simulink model "TST_PthLead_TrqCalc"  (R2016b)
settings: Solver=FixedStepDiscrete  StartTime=0.0  StopTime=simTime  FixedStep=sampleTime  RelTol=1e-3
values from neighbouring files (symbols this model uses):
  testCase = 1    [initTST_PthLead_TrqCalc_001.m]    (also in initTST_PthLead_TrqCalc_002.m = 2; initTST_PthLead_TrqCalc_003.m = 3)
libraries: simulink x13, UnitTest_Lib x9
settings Model: Creator=zhengjinyan  LastModifiedBy=zhengjinyan
settings DebuggingCC: SignalRangeChecking=error

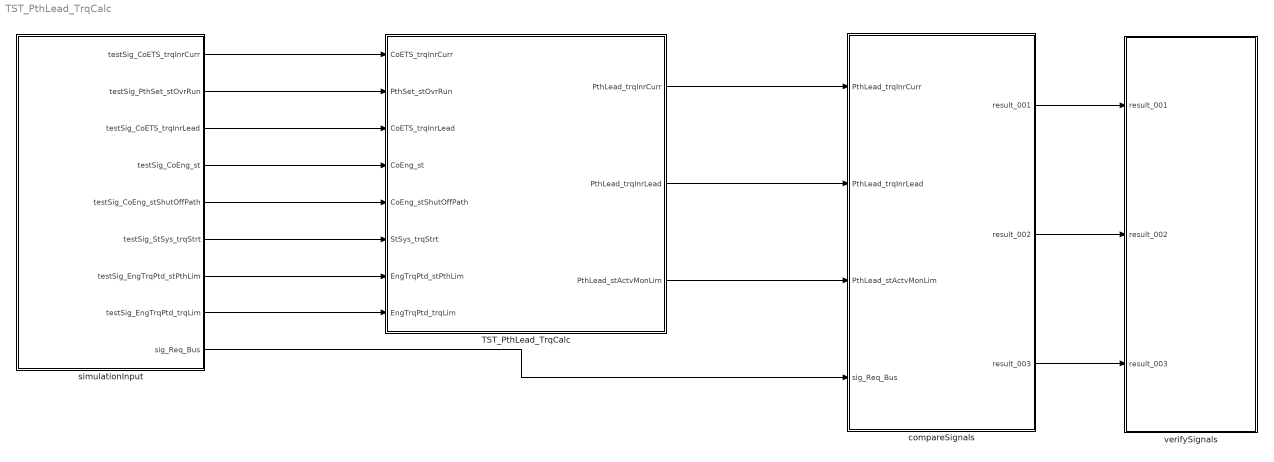
== system TST_PthLead_TrqCalc ==
  TST_PthLead_TrqCalc : Subsystem
  compareSignals : Subsystem
  simulationInput : Subsystem
  verifySignals : Subsystem
  wires:
  simulationInput/1(testSig_CoETS_trqInrCurr) -> TST_PthLead_TrqCalc/1(CoETS_trqInrCurr)
  simulationInput/2(testSig_PthSet_stOvrRun) -> TST_PthLead_TrqCalc/2(PthSet_stOvrRun)
  simulationInput/3(testSig_CoETS_trqInrLead) -> TST_PthLead_TrqCalc/3(CoETS_trqInrLead)
  simulationInput/4(testSig_CoEng_st) -> TST_PthLead_TrqCalc/4(CoEng_st)
  simulationInput/5(testSig_CoEng_stShutOffPath) -> TST_PthLead_TrqCalc/5(CoEng_stShutOffPath)
  simulationInput/6(testSig_StSys_trqStrt) -> TST_PthLead_TrqCalc/6(StSys_trqStrt)
  simulationInput/7(testSig_EngTrqPtd_stPthLim) -> TST_PthLead_TrqCalc/7(EngTrqPtd_stPthLim)
  simulationInput/8(testSig_EngTrqPtd_trqLim) -> TST_PthLead_TrqCalc/8(EngTrqPtd_trqLim)
  TST_PthLead_TrqCalc/1(PthLead_trqInrCurr) -> compareSignals/1(PthLead_trqInrCurr)
  TST_PthLead_TrqCalc/2(PthLead_trqInrLead) -> compareSignals/2(PthLead_trqInrLead)
  TST_PthLead_TrqCalc/3(PthLead_stActvMonLim) -> compareSignals/3(PthLead_stActvMonLim)
  simulationInput/9(sig_Req_Bus) -> compareSignals/4(sig_Req_Bus)
  compareSignals/1(result_001) -> verifySignals/1(result_001)
  compareSignals/2(result_002) -> verifySignals/2(result_002)
  compareSignals/3(result_003) -> verifySignals/3(result_003)

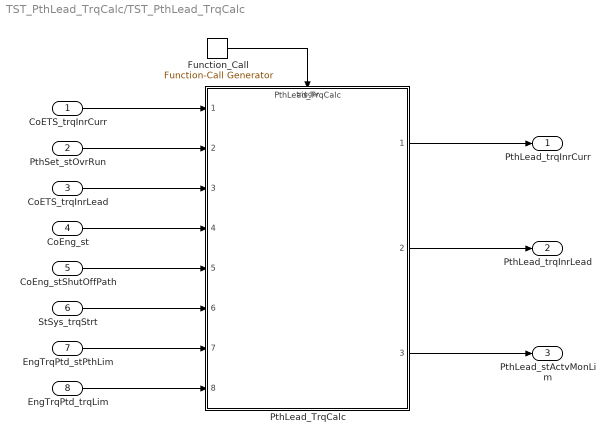
== system TST_PthLead_TrqCalc/TST_PthLead_TrqCalc ==
  CoETS_trqInrCurr : Inport
  PthSet_stOvrRun : Inport  Port=2
  CoETS_trqInrLead : Inport  Port=3
  CoEng_st : Inport  Port=4
  CoEng_stShutOffPath : Inport  Port=5
  StSys_trqStrt : Inport  Port=6
  EngTrqPtd_stPthLim : Inport  Port=7
  EngTrqPtd_trqLim : Inport  Port=8
  Function_Call : simulink/Ports & Subsystems/Function-Call Generator  sample_time=sampleTime  numberOfIterations=1
  PthLead_TrqCalc : ModelReference  ModelNameDialog=PthLead_TrqCalc  SimulationMode=Normal  ModelReferenceVersion=1.4  TriggerPortName=function  TriggerPortTriggerType=function-call  TriggerPortStatesWhenEnabling=held
  PthLead_trqInrCurr : Outport
  PthLead_trqInrLead : Outport  Port=2
  PthLead_stActvMonLim : Outport  Port=3
  wires:
  Function_Call/1 -> PthLead_TrqCalc/Trigger
  CoETS_trqInrCurr/1 -> PthLead_TrqCalc/1
  PthSet_stOvrRun/1 -> PthLead_TrqCalc/2
  CoETS_trqInrLead/1 -> PthLead_TrqCalc/3
  CoEng_st/1 -> PthLead_TrqCalc/4
  CoEng_stShutOffPath/1 -> PthLead_TrqCalc/5
  StSys_trqStrt/1 -> PthLead_TrqCalc/6
  EngTrqPtd_stPthLim/1 -> PthLead_TrqCalc/7
  EngTrqPtd_trqLim/1 -> PthLead_TrqCalc/8
  PthLead_TrqCalc/1 -> PthLead_trqInrCurr/1
  PthLead_TrqCalc/2 -> PthLead_trqInrLead/1
  PthLead_TrqCalc/3 -> PthLead_stActvMonLim/1

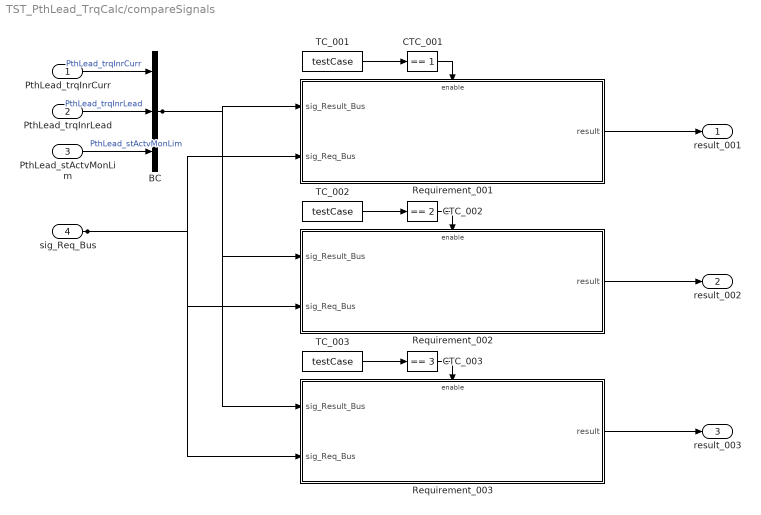
== system TST_PthLead_TrqCalc/compareSignals ==
  PthLead_trqInrCurr : Inport
  PthLead_trqInrLead : Inport  Port=2
  PthLead_stActvMonLim : Inport  Port=3
  sig_Req_Bus : Inport  Port=4
  BC : BusCreator  Inputs=3
  CTC_001 : simulink/Logic and Bit Operations/Compare To Constant  relop===  const=1  OutDataTypeStr=boolean
  CTC_002 : simulink/Logic and Bit Operations/Compare To Constant  relop===  const=2  OutDataTypeStr=boolean
  CTC_003 : simulink/Logic and Bit Operations/Compare To Constant  relop===  const=3  OutDataTypeStr=boolean
  Requirement_001 : Subsystem
  Requirement_002 : Subsystem
  Requirement_003 : Subsystem
  TC_001 : Constant  Value=testCase
  TC_002 : Constant  Value=testCase
  TC_003 : Constant  Value=testCase
  result_001 : Outport
  result_002 : Outport  Port=2
  result_003 : Outport  Port=3
  wires:
  PthLead_trqInrCurr/1 -> BC/1  "PthLead_trqInrCurr"
  PthLead_trqInrLead/1 -> BC/2  "PthLead_trqInrLead"
  PthLead_stActvMonLim/1 -> BC/3  "PthLead_stActvMonLim"
  TC_001/1 -> CTC_001/1
  CTC_001/1 -> Requirement_001/Enable
  sig_Req_Bus/1 -> Requirement_001/2(sig_Req_Bus), Requirement_002/2(sig_Req_Bus), Requirement_003/2(sig_Req_Bus)
  BC/1 -> Requirement_001/1(sig_Result_Bus), Requirement_002/1(sig_Result_Bus), Requirement_003/1(sig_Result_Bus)
  Requirement_001/1(result) -> result_001/1
  TC_002/1 -> CTC_002/1
  CTC_002/1 -> Requirement_002/Enable
  Requirement_002/1(result) -> result_002/1
  TC_003/1 -> CTC_003/1
  CTC_003/1 -> Requirement_003/Enable
  Requirement_003/1(result) -> result_003/1

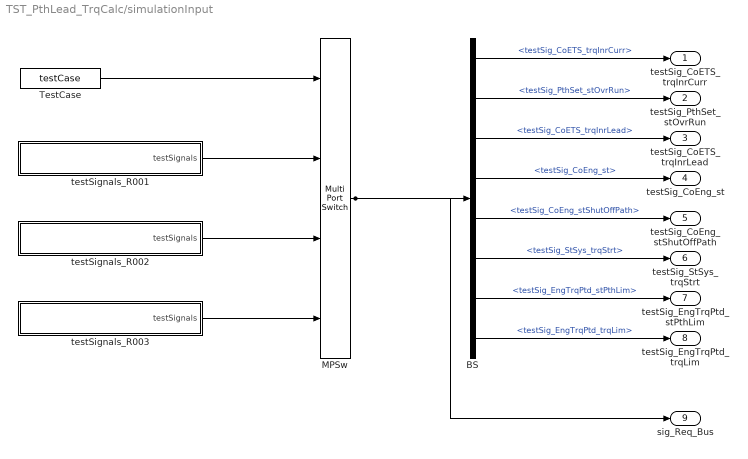
== system TST_PthLead_TrqCalc/simulationInput ==
  BS : BusSelector  OutputSignals=testSig_CoETS_trqInrCurr,testSig_PthSet_stOvrRun,testSig_CoETS_trqInrLead,testSig_CoEng_st,testSig_CoEng_stShutOffPath,testSig_StSys_trqStrt,testSig_EngTrqPtd_stPthLim,testSig_EngTrqPtd_trqLim
  MPSw : MultiPortSwitch  SaturateOnIntegerOverflow=on  InputSameDT=on
  TestCase : Constant  Value=testCase
  testSignals_R001 : Subsystem
  testSignals_R002 : Subsystem
  testSignals_R003 : Subsystem
  testSig_CoETS_trqInrCurr : Outport
  testSig_PthSet_stOvrRun : Outport  Port=2
  testSig_CoETS_trqInrLead : Outport  Port=3
  testSig_CoEng_st : Outport  Port=4
  testSig_CoEng_stShutOffPath : Outport  Port=5
  testSig_StSys_trqStrt : Outport  Port=6
  testSig_EngTrqPtd_stPthLim : Outport  Port=7
  testSig_EngTrqPtd_trqLim : Outport  Port=8
  sig_Req_Bus : Outport  Port=9
  wires:
  BS/1 -> testSig_CoETS_trqInrCurr/1  "<testSig_CoETS_trqInrCurr>"
  BS/2 -> testSig_PthSet_stOvrRun/1  "<testSig_PthSet_stOvrRun>"
  BS/3 -> testSig_CoETS_trqInrLead/1  "<testSig_CoETS_trqInrLead>"
  BS/4 -> testSig_CoEng_st/1  "<testSig_CoEng_st>"
  BS/5 -> testSig_CoEng_stShutOffPath/1  "<testSig_CoEng_stShutOffPath>"
  BS/6 -> testSig_StSys_trqStrt/1  "<testSig_StSys_trqStrt>"
  BS/7 -> testSig_EngTrqPtd_stPthLim/1  "<testSig_EngTrqPtd_stPthLim>"
  BS/8 -> testSig_EngTrqPtd_trqLim/1  "<testSig_EngTrqPtd_trqLim>"
  MPSw/1 -> BS/1, sig_Req_Bus/1
  TestCase/1 -> MPSw/1
  testSignals_R001/1(testSignals) -> MPSw/2
  testSignals_R002/1(testSignals) -> MPSw/3
  testSignals_R003/1(testSignals) -> MPSw/4

== system TST_PthLead_TrqCalc/verifySignals ==
  result_001 : Inport
  result_002 : Inport  Port=2
  result_003 : Inport  Port=3
  Assertion_001 : Assertion  Enabled=off
  Assertion_002 : Assertion  Enabled=off
  Assertion_003 : Assertion  Enabled=off
  wires:
  result_001/1 -> Assertion_001/1
  result_002/1 -> Assertion_002/1
  result_003/1 -> Assertion_003/1

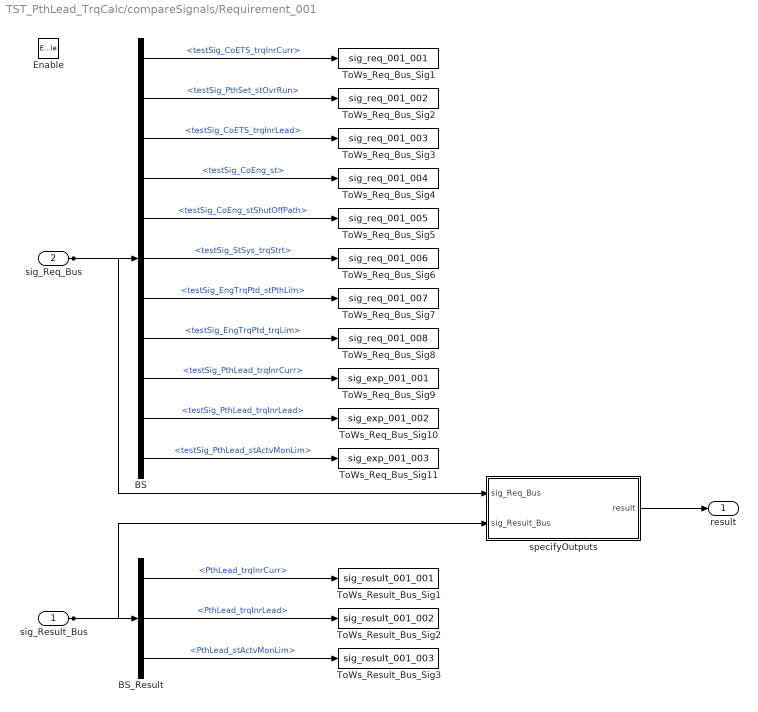
== system TST_PthLead_TrqCalc/compareSignals/Requirement_001 ==
  sig_Result_Bus : Inport
  sig_Req_Bus : Inport  Port=2
  Enable : EnablePort
  BS : BusSelector  OutputSignals=testSig_CoETS_trqInrCurr,testSig_PthSet_stOvrRun,testSig_CoETS_trqInrLead,testSig_CoEng_st,testSig_CoEng_stShutOffPath,testSig_StSys_trqStrt,testSig_EngTrqPtd_stPthLim,testSig_EngTrqPtd_trqLim,testSig_PthLead_trqInrCurr,testSig_PthLead_trqInrLead,testSig_PthLead_stActvMonLim
  BS_Result : BusSelector  OutputSignals=PthLead_trqInrCurr,PthLead_trqInrLead,PthLead_stActvMonLim
  ToWs_Req_Bus_Sig1 : ToWorkspace  VariableName=sig_req_001_001  SaveFormat=Structure With Time
  ToWs_Req_Bus_Sig10 : ToWorkspace  VariableName=sig_exp_001_002  SaveFormat=Structure With Time
  ToWs_Req_Bus_Sig11 : ToWorkspace  VariableName=sig_exp_001_003  SaveFormat=Structure With Time
  ToWs_Req_Bus_Sig2 : ToWorkspace  VariableName=sig_req_001_002  SaveFormat=Structure With Time
  ToWs_Req_Bus_Sig3 : ToWorkspace  VariableName=sig_req_001_003  SaveFormat=Structure With Time
  ToWs_Req_Bus_Sig4 : ToWorkspace  VariableName=sig_req_001_004  SaveFormat=Structure With Time
  ToWs_Req_Bus_Sig5 : ToWorkspace  VariableName=sig_req_001_005  SaveFormat=Structure With Time
  ToWs_Req_Bus_Sig6 : ToWorkspace  VariableName=sig_req_001_006  SaveFormat=Structure With Time
  ToWs_Req_Bus_Sig7 : ToWorkspace  VariableName=sig_req_001_007  SaveFormat=Structure With Time
  ToWs_Req_Bus_Sig8 : ToWorkspace  VariableName=sig_req_001_008  SaveFormat=Structure With Time
  ToWs_Req_Bus_Sig9 : ToWorkspace  VariableName=sig_exp_001_001  SaveFormat=Structure With Time
  ToWs_Result_Bus_Sig1 : ToWorkspace  VariableName=sig_result_001_001  SaveFormat=Structure With Time
  ToWs_Result_Bus_Sig2 : ToWorkspace  VariableName=sig_result_001_002  SaveFormat=Structure With Time
  ToWs_Result_Bus_Sig3 : ToWorkspace  VariableName=sig_result_001_003  SaveFormat=Structure With Time
  specifyOutputs : Subsystem
  result : Outport
  wires:
  sig_Req_Bus/1 -> BS/1, specifyOutputs/1(sig_Req_Bus)
  BS/1 -> ToWs_Req_Bus_Sig1/1  "<testSig_CoETS_trqInrCurr>"
  BS/2 -> ToWs_Req_Bus_Sig2/1  "<testSig_PthSet_stOvrRun>"
  BS/3 -> ToWs_Req_Bus_Sig3/1  "<testSig_CoETS_trqInrLead>"
  BS/4 -> ToWs_Req_Bus_Sig4/1  "<testSig_CoEng_st>"
  BS/5 -> ToWs_Req_Bus_Sig5/1  "<testSig_CoEng_stShutOffPath>"
  BS/6 -> ToWs_Req_Bus_Sig6/1  "<testSig_StSys_trqStrt>"
  BS/7 -> ToWs_Req_Bus_Sig7/1  "<testSig_EngTrqPtd_stPthLim>"
  BS/8 -> ToWs_Req_Bus_Sig8/1  "<testSig_EngTrqPtd_trqLim>"
  BS/9 -> ToWs_Req_Bus_Sig9/1  "<testSig_PthLead_trqInrCurr>"
  BS/10 -> ToWs_Req_Bus_Sig10/1  "<testSig_PthLead_trqInrLead>"
  BS/11 -> ToWs_Req_Bus_Sig11/1  "<testSig_PthLead_stActvMonLim>"
  sig_Result_Bus/1 -> BS_Result/1, specifyOutputs/2(sig_Result_Bus)
  BS_Result/1 -> ToWs_Result_Bus_Sig1/1  "<PthLead_trqInrCurr>"
  BS_Result/2 -> ToWs_Result_Bus_Sig2/1  "<PthLead_trqInrLead>"
  BS_Result/3 -> ToWs_Result_Bus_Sig3/1  "<PthLead_stActvMonLim>"
  specifyOutputs/1(result) -> result/1

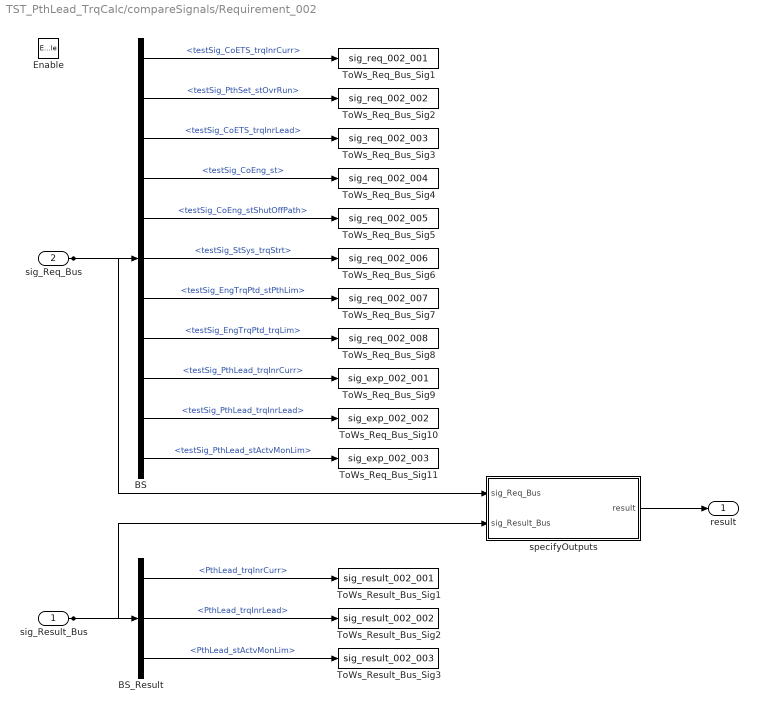
== system TST_PthLead_TrqCalc/compareSignals/Requirement_002 ==
  sig_Result_Bus : Inport
  sig_Req_Bus : Inport  Port=2
  Enable : EnablePort
  BS : BusSelector  OutputSignals=testSig_CoETS_trqInrCurr,testSig_PthSet_stOvrRun,testSig_CoETS_trqInrLead,testSig_CoEng_st,testSig_CoEng_stShutOffPath,testSig_StSys_trqStrt,testSig_EngTrqPtd_stPthLim,testSig_EngTrqPtd_trqLim,testSig_PthLead_trqInrCurr,testSig_PthLead_trqInrLead,testSig_PthLead_stActvMonLim
  BS_Result : BusSelector  OutputSignals=PthLead_trqInrCurr,PthLead_trqInrLead,PthLead_stActvMonLim
  ToWs_Req_Bus_Sig1 : ToWorkspace  VariableName=sig_req_002_001  SaveFormat=Structure With Time
  ToWs_Req_Bus_Sig10 : ToWorkspace  VariableName=sig_exp_002_002  SaveFormat=Structure With Time
  ToWs_Req_Bus_Sig11 : ToWorkspace  VariableName=sig_exp_002_003  SaveFormat=Structure With Time
  ToWs_Req_Bus_Sig2 : ToWorkspace  VariableName=sig_req_002_002  SaveFormat=Structure With Time
  ToWs_Req_Bus_Sig3 : ToWorkspace  VariableName=sig_req_002_003  SaveFormat=Structure With Time
  ToWs_Req_Bus_Sig4 : ToWorkspace  VariableName=sig_req_002_004  SaveFormat=Structure With Time
  ToWs_Req_Bus_Sig5 : ToWorkspace  VariableName=sig_req_002_005  SaveFormat=Structure With Time
  ToWs_Req_Bus_Sig6 : ToWorkspace  VariableName=sig_req_002_006  SaveFormat=Structure With Time
  ToWs_Req_Bus_Sig7 : ToWorkspace  VariableName=sig_req_002_007  SaveFormat=Structure With Time
  ToWs_Req_Bus_Sig8 : ToWorkspace  VariableName=sig_req_002_008  SaveFormat=Structure With Time
  ToWs_Req_Bus_Sig9 : ToWorkspace  VariableName=sig_exp_002_001  SaveFormat=Structure With Time
  ToWs_Result_Bus_Sig1 : ToWorkspace  VariableName=sig_result_002_001  SaveFormat=Structure With Time
  ToWs_Result_Bus_Sig2 : ToWorkspace  VariableName=sig_result_002_002  SaveFormat=Structure With Time
  ToWs_Result_Bus_Sig3 : ToWorkspace  VariableName=sig_result_002_003  SaveFormat=Structure With Time
  specifyOutputs : Subsystem
  result : Outport
  wires:
  sig_Req_Bus/1 -> BS/1, specifyOutputs/1(sig_Req_Bus)
  BS/1 -> ToWs_Req_Bus_Sig1/1  "<testSig_CoETS_trqInrCurr>"
  BS/2 -> ToWs_Req_Bus_Sig2/1  "<testSig_PthSet_stOvrRun>"
  BS/3 -> ToWs_Req_Bus_Sig3/1  "<testSig_CoETS_trqInrLead>"
  BS/4 -> ToWs_Req_Bus_Sig4/1  "<testSig_CoEng_st>"
  BS/5 -> ToWs_Req_Bus_Sig5/1  "<testSig_CoEng_stShutOffPath>"
  BS/6 -> ToWs_Req_Bus_Sig6/1  "<testSig_StSys_trqStrt>"
  BS/7 -> ToWs_Req_Bus_Sig7/1  "<testSig_EngTrqPtd_stPthLim>"
  BS/8 -> ToWs_Req_Bus_Sig8/1  "<testSig_EngTrqPtd_trqLim>"
  BS/9 -> ToWs_Req_Bus_Sig9/1  "<testSig_PthLead_trqInrCurr>"
  BS/10 -> ToWs_Req_Bus_Sig10/1  "<testSig_PthLead_trqInrLead>"
  BS/11 -> ToWs_Req_Bus_Sig11/1  "<testSig_PthLead_stActvMonLim>"
  sig_Result_Bus/1 -> BS_Result/1, specifyOutputs/2(sig_Result_Bus)
  BS_Result/1 -> ToWs_Result_Bus_Sig1/1  "<PthLead_trqInrCurr>"
  BS_Result/2 -> ToWs_Result_Bus_Sig2/1  "<PthLead_trqInrLead>"
  BS_Result/3 -> ToWs_Result_Bus_Sig3/1  "<PthLead_stActvMonLim>"
  specifyOutputs/1(result) -> result/1

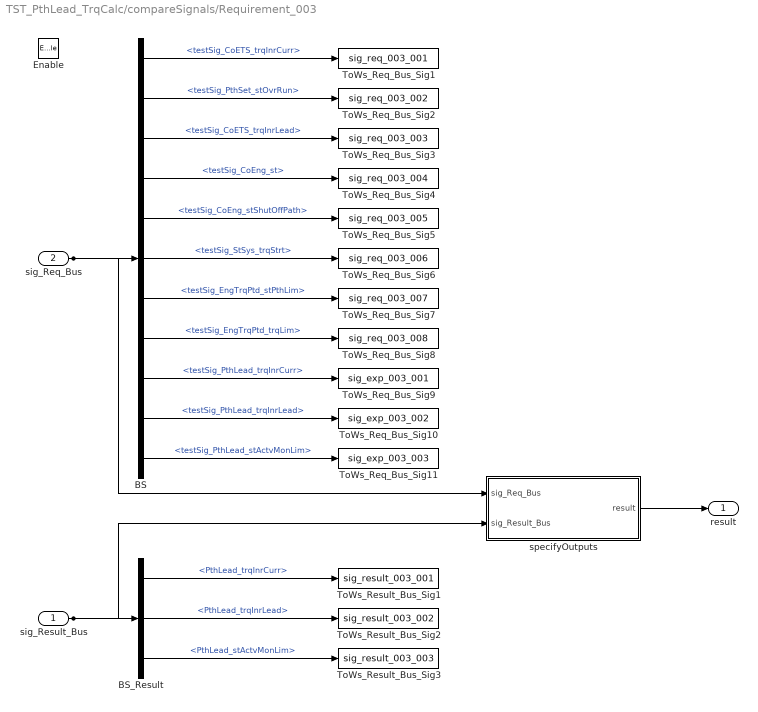
== system TST_PthLead_TrqCalc/compareSignals/Requirement_003 ==
  sig_Result_Bus : Inport
  sig_Req_Bus : Inport  Port=2
  Enable : EnablePort
  BS : BusSelector  OutputSignals=testSig_CoETS_trqInrCurr,testSig_PthSet_stOvrRun,testSig_CoETS_trqInrLead,testSig_CoEng_st,testSig_CoEng_stShutOffPath,testSig_StSys_trqStrt,testSig_EngTrqPtd_stPthLim,testSig_EngTrqPtd_trqLim,testSig_PthLead_trqInrCurr,testSig_PthLead_trqInrLead,testSig_PthLead_stActvMonLim
  BS_Result : BusSelector  OutputSignals=PthLead_trqInrCurr,PthLead_trqInrLead,PthLead_stActvMonLim
  ToWs_Req_Bus_Sig1 : ToWorkspace  VariableName=sig_req_003_001  SaveFormat=Structure With Time
  ToWs_Req_Bus_Sig10 : ToWorkspace  VariableName=sig_exp_003_002  SaveFormat=Structure With Time
  ToWs_Req_Bus_Sig11 : ToWorkspace  VariableName=sig_exp_003_003  SaveFormat=Structure With Time
  ToWs_Req_Bus_Sig2 : ToWorkspace  VariableName=sig_req_003_002  SaveFormat=Structure With Time
  ToWs_Req_Bus_Sig3 : ToWorkspace  VariableName=sig_req_003_003  SaveFormat=Structure With Time
  ToWs_Req_Bus_Sig4 : ToWorkspace  VariableName=sig_req_003_004  SaveFormat=Structure With Time
  ToWs_Req_Bus_Sig5 : ToWorkspace  VariableName=sig_req_003_005  SaveFormat=Structure With Time
  ToWs_Req_Bus_Sig6 : ToWorkspace  VariableName=sig_req_003_006  SaveFormat=Structure With Time
  ToWs_Req_Bus_Sig7 : ToWorkspace  VariableName=sig_req_003_007  SaveFormat=Structure With Time
  ToWs_Req_Bus_Sig8 : ToWorkspace  VariableName=sig_req_003_008  SaveFormat=Structure With Time
  ToWs_Req_Bus_Sig9 : ToWorkspace  VariableName=sig_exp_003_001  SaveFormat=Structure With Time
  ToWs_Result_Bus_Sig1 : ToWorkspace  VariableName=sig_result_003_001  SaveFormat=Structure With Time
  ToWs_Result_Bus_Sig2 : ToWorkspace  VariableName=sig_result_003_002  SaveFormat=Structure With Time
  ToWs_Result_Bus_Sig3 : ToWorkspace  VariableName=sig_result_003_003  SaveFormat=Structure With Time
  specifyOutputs : Subsystem
  result : Outport
  wires:
  sig_Req_Bus/1 -> BS/1, specifyOutputs/1(sig_Req_Bus)
  BS/1 -> ToWs_Req_Bus_Sig1/1  "<testSig_CoETS_trqInrCurr>"
  BS/2 -> ToWs_Req_Bus_Sig2/1  "<testSig_PthSet_stOvrRun>"
  BS/3 -> ToWs_Req_Bus_Sig3/1  "<testSig_CoETS_trqInrLead>"
  BS/4 -> ToWs_Req_Bus_Sig4/1  "<testSig_CoEng_st>"
  BS/5 -> ToWs_Req_Bus_Sig5/1  "<testSig_CoEng_stShutOffPath>"
  BS/6 -> ToWs_Req_Bus_Sig6/1  "<testSig_StSys_trqStrt>"
  BS/7 -> ToWs_Req_Bus_Sig7/1  "<testSig_EngTrqPtd_stPthLim>"
  BS/8 -> ToWs_Req_Bus_Sig8/1  "<testSig_EngTrqPtd_trqLim>"
  BS/9 -> ToWs_Req_Bus_Sig9/1  "<testSig_PthLead_trqInrCurr>"
  BS/10 -> ToWs_Req_Bus_Sig10/1  "<testSig_PthLead_trqInrLead>"
  BS/11 -> ToWs_Req_Bus_Sig11/1  "<testSig_PthLead_stActvMonLim>"
  sig_Result_Bus/1 -> BS_Result/1, specifyOutputs/2(sig_Result_Bus)
  BS_Result/1 -> ToWs_Result_Bus_Sig1/1  "<PthLead_trqInrCurr>"
  BS_Result/2 -> ToWs_Result_Bus_Sig2/1  "<PthLead_trqInrLead>"
  BS_Result/3 -> ToWs_Result_Bus_Sig3/1  "<PthLead_stActvMonLim>"
  specifyOutputs/1(result) -> result/1

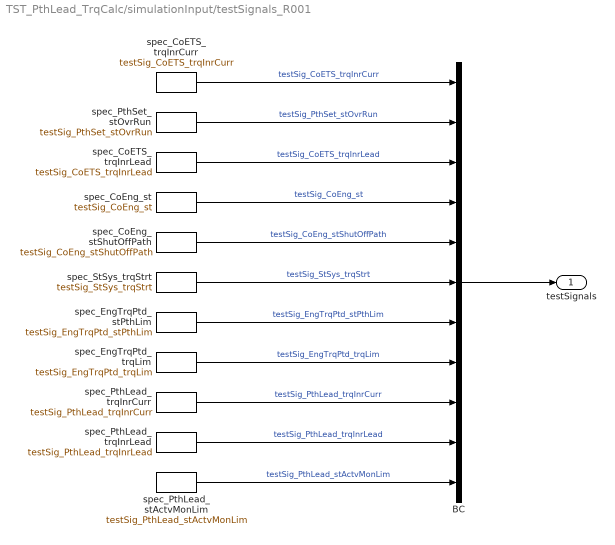
== system TST_PthLead_TrqCalc/simulationInput/testSignals_R001 ==
  BC : BusCreator  Inputs=11
  spec_CoETS_trqInrCurr : FromWorkspace  VariableName=testSig_CoETS_trqInrCurr  Interpolate=off  OutputAfterFinalValue=Holding final value
  spec_CoETS_trqInrLead : FromWorkspace  VariableName=testSig_CoETS_trqInrLead  Interpolate=off  OutputAfterFinalValue=Holding final value
  spec_CoEng_st : FromWorkspace  VariableName=testSig_CoEng_st  Interpolate=off  OutputAfterFinalValue=Holding final value
  spec_CoEng_stShutOffPath : FromWorkspace  VariableName=testSig_CoEng_stShutOffPath  Interpolate=off  OutputAfterFinalValue=Holding final value
  spec_EngTrqPtd_stPthLim : FromWorkspace  VariableName=testSig_EngTrqPtd_stPthLim  Interpolate=off  OutputAfterFinalValue=Holding final value
  spec_EngTrqPtd_trqLim : FromWorkspace  VariableName=testSig_EngTrqPtd_trqLim  Interpolate=off  OutputAfterFinalValue=Holding final value
  spec_PthLead_stActvMonLim : FromWorkspace  VariableName=testSig_PthLead_stActvMonLim  Interpolate=off  OutputAfterFinalValue=Holding final value
  spec_PthLead_trqInrCurr : FromWorkspace  VariableName=testSig_PthLead_trqInrCurr  Interpolate=off  OutputAfterFinalValue=Holding final value
  spec_PthLead_trqInrLead : FromWorkspace  VariableName=testSig_PthLead_trqInrLead  Interpolate=off  OutputAfterFinalValue=Holding final value
  spec_PthSet_stOvrRun : FromWorkspace  VariableName=testSig_PthSet_stOvrRun  Interpolate=off  OutputAfterFinalValue=Holding final value
  spec_StSys_trqStrt : FromWorkspace  VariableName=testSig_StSys_trqStrt  Interpolate=off  OutputAfterFinalValue=Holding final value
  testSignals : Outport
  wires:
  BC/1 -> testSignals/1
  spec_CoETS_trqInrCurr/1 -> BC/1  "testSig_CoETS_trqInrCurr"
  spec_PthSet_stOvrRun/1 -> BC/2  "testSig_PthSet_stOvrRun"
  spec_CoETS_trqInrLead/1 -> BC/3  "testSig_CoETS_trqInrLead"
  spec_CoEng_st/1 -> BC/4  "testSig_CoEng_st"
  spec_CoEng_stShutOffPath/1 -> BC/5  "testSig_CoEng_stShutOffPath"
  spec_StSys_trqStrt/1 -> BC/6  "testSig_StSys_trqStrt"
  spec_EngTrqPtd_stPthLim/1 -> BC/7  "testSig_EngTrqPtd_stPthLim"
  spec_EngTrqPtd_trqLim/1 -> BC/8  "testSig_EngTrqPtd_trqLim"
  spec_PthLead_trqInrCurr/1 -> BC/9  "testSig_PthLead_trqInrCurr"
  spec_PthLead_trqInrLead/1 -> BC/10  "testSig_PthLead_trqInrLead"
  spec_PthLead_stActvMonLim/1 -> BC/11  "testSig_PthLead_stActvMonLim"

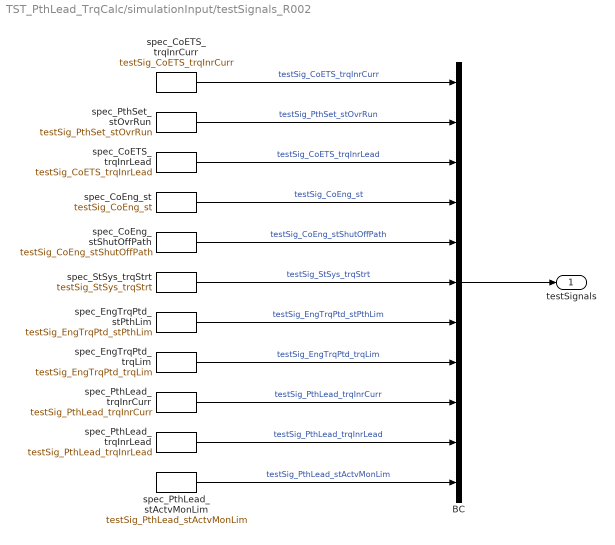
== system TST_PthLead_TrqCalc/simulationInput/testSignals_R002 ==
  BC : BusCreator  Inputs=11
  spec_CoETS_trqInrCurr : FromWorkspace  VariableName=testSig_CoETS_trqInrCurr  Interpolate=off  OutputAfterFinalValue=Holding final value
  spec_CoETS_trqInrLead : FromWorkspace  VariableName=testSig_CoETS_trqInrLead  Interpolate=off  OutputAfterFinalValue=Holding final value
  spec_CoEng_st : FromWorkspace  VariableName=testSig_CoEng_st  Interpolate=off  OutputAfterFinalValue=Holding final value
  spec_CoEng_stShutOffPath : FromWorkspace  VariableName=testSig_CoEng_stShutOffPath  Interpolate=off  OutputAfterFinalValue=Holding final value
  spec_EngTrqPtd_stPthLim : FromWorkspace  VariableName=testSig_EngTrqPtd_stPthLim  Interpolate=off  OutputAfterFinalValue=Holding final value
  spec_EngTrqPtd_trqLim : FromWorkspace  VariableName=testSig_EngTrqPtd_trqLim  Interpolate=off  OutputAfterFinalValue=Holding final value
  spec_PthLead_stActvMonLim : FromWorkspace  VariableName=testSig_PthLead_stActvMonLim  Interpolate=off  OutputAfterFinalValue=Holding final value
  spec_PthLead_trqInrCurr : FromWorkspace  VariableName=testSig_PthLead_trqInrCurr  Interpolate=off  OutputAfterFinalValue=Holding final value
  spec_PthLead_trqInrLead : FromWorkspace  VariableName=testSig_PthLead_trqInrLead  Interpolate=off  OutputAfterFinalValue=Holding final value
  spec_PthSet_stOvrRun : FromWorkspace  VariableName=testSig_PthSet_stOvrRun  Interpolate=off  OutputAfterFinalValue=Holding final value
  spec_StSys_trqStrt : FromWorkspace  VariableName=testSig_StSys_trqStrt  Interpolate=off  OutputAfterFinalValue=Holding final value
  testSignals : Outport
  wires:
  BC/1 -> testSignals/1
  spec_CoETS_trqInrCurr/1 -> BC/1  "testSig_CoETS_trqInrCurr"
  spec_PthSet_stOvrRun/1 -> BC/2  "testSig_PthSet_stOvrRun"
  spec_CoETS_trqInrLead/1 -> BC/3  "testSig_CoETS_trqInrLead"
  spec_CoEng_st/1 -> BC/4  "testSig_CoEng_st"
  spec_CoEng_stShutOffPath/1 -> BC/5  "testSig_CoEng_stShutOffPath"
  spec_StSys_trqStrt/1 -> BC/6  "testSig_StSys_trqStrt"
  spec_EngTrqPtd_stPthLim/1 -> BC/7  "testSig_EngTrqPtd_stPthLim"
  spec_EngTrqPtd_trqLim/1 -> BC/8  "testSig_EngTrqPtd_trqLim"
  spec_PthLead_trqInrCurr/1 -> BC/9  "testSig_PthLead_trqInrCurr"
  spec_PthLead_trqInrLead/1 -> BC/10  "testSig_PthLead_trqInrLead"
  spec_PthLead_stActvMonLim/1 -> BC/11  "testSig_PthLead_stActvMonLim"

== system TST_PthLead_TrqCalc/simulationInput/testSignals_R003 ==
  BC : BusCreator  Inputs=11
  spec_CoETS_trqInrCurr : FromWorkspace  VariableName=testSig_CoETS_trqInrCurr  Interpolate=off  OutputAfterFinalValue=Holding final value
  spec_CoETS_trqInrLead : FromWorkspace  VariableName=testSig_CoETS_trqInrLead  Interpolate=off  OutputAfterFinalValue=Holding final value
  spec_CoEng_st : FromWorkspace  VariableName=testSig_CoEng_st  Interpolate=off  OutputAfterFinalValue=Holding final value
  spec_CoEng_stShutOffPath : FromWorkspace  VariableName=testSig_CoEng_stShutOffPath  Interpolate=off  OutputAfterFinalValue=Holding final value
  spec_EngTrqPtd_stPthLim : FromWorkspace  VariableName=testSig_EngTrqPtd_stPthLim  Interpolate=off  OutputAfterFinalValue=Holding final value
  spec_EngTrqPtd_trqLim : FromWorkspace  VariableName=testSig_EngTrqPtd_trqLim  Interpolate=off  OutputAfterFinalValue=Holding final value
  spec_PthLead_stActvMonLim : FromWorkspace  VariableName=testSig_PthLead_stActvMonLim  Interpolate=off  OutputAfterFinalValue=Holding final value
  spec_PthLead_trqInrCurr : FromWorkspace  VariableName=testSig_PthLead_trqInrCurr  Interpolate=off  OutputAfterFinalValue=Holding final value
  spec_PthLead_trqInrLead : FromWorkspace  VariableName=testSig_PthLead_trqInrLead  Interpolate=off  OutputAfterFinalValue=Holding final value
  spec_PthSet_stOvrRun : FromWorkspace  VariableName=testSig_PthSet_stOvrRun  Interpolate=off  OutputAfterFinalValue=Holding final value
  spec_StSys_trqStrt : FromWorkspace  VariableName=testSig_StSys_trqStrt  Interpolate=off  OutputAfterFinalValue=Holding final value
  testSignals : Outport
  wires:
  BC/1 -> testSignals/1
  spec_CoETS_trqInrCurr/1 -> BC/1  "testSig_CoETS_trqInrCurr"
  spec_PthSet_stOvrRun/1 -> BC/2  "testSig_PthSet_stOvrRun"
  spec_CoETS_trqInrLead/1 -> BC/3  "testSig_CoETS_trqInrLead"
  spec_CoEng_st/1 -> BC/4  "testSig_CoEng_st"
  spec_CoEng_stShutOffPath/1 -> BC/5  "testSig_CoEng_stShutOffPath"
  spec_StSys_trqStrt/1 -> BC/6  "testSig_StSys_trqStrt"
  spec_EngTrqPtd_stPthLim/1 -> BC/7  "testSig_EngTrqPtd_stPthLim"
  spec_EngTrqPtd_trqLim/1 -> BC/8  "testSig_EngTrqPtd_trqLim"
  spec_PthLead_trqInrCurr/1 -> BC/9  "testSig_PthLead_trqInrCurr"
  spec_PthLead_trqInrLead/1 -> BC/10  "testSig_PthLead_trqInrLead"
  spec_PthLead_stActvMonLim/1 -> BC/11  "testSig_PthLead_stActvMonLim"

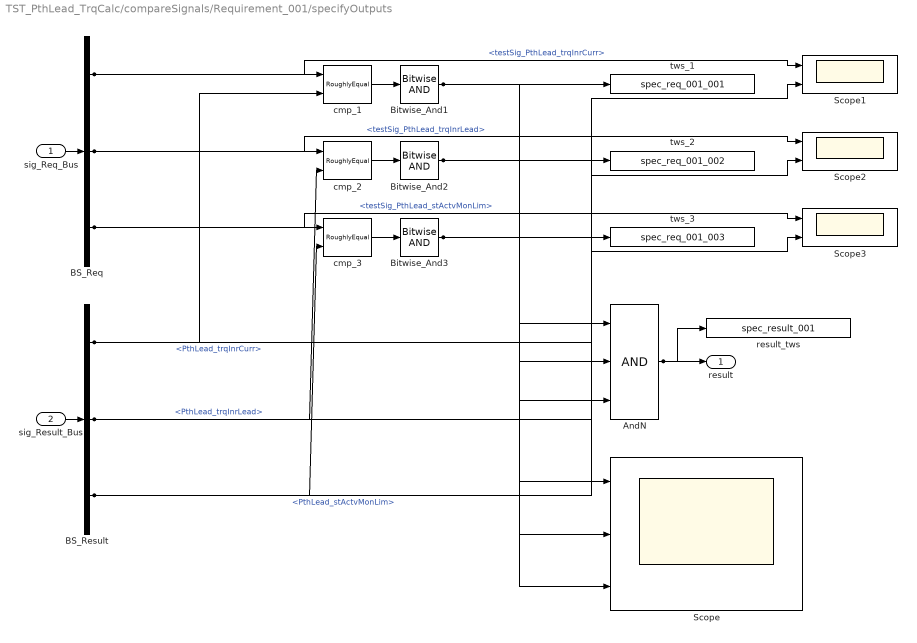
== system TST_PthLead_TrqCalc/compareSignals/Requirement_001/specifyOutputs ==
  sig_Req_Bus : Inport
  sig_Result_Bus : Inport  Port=2
  AndN : Logic  Inputs=3
  BS_Req : BusSelector  OutputSignals=testSig_PthLead_trqInrCurr,testSig_PthLead_trqInrLead,testSig_PthLead_stActvMonLim
  BS_Result : BusSelector  OutputSignals=PthLead_trqInrCurr,PthLead_trqInrLead,PthLead_stActvMonLim
  Bitwise_And1 : simulink/Logic and Bit Operations/Bitwise Operator  logicop=AND  UseBitMask=off  BitMask=bin2dec('11011001')  BitMaskRealWorld=Stored Integer
  Bitwise_And2 : simulink/Logic and Bit Operations/Bitwise Operator  logicop=AND  UseBitMask=off  BitMask=bin2dec('11011001')  BitMaskRealWorld=Stored Integer
  Bitwise_And3 : simulink/Logic and Bit Operations/Bitwise Operator  logicop=AND  UseBitMask=off  BitMask=bin2dec('11011001')  BitMaskRealWorld=Stored Integer
  Scope : Scope  NumInputPorts=3
  Scope1 : Scope  NumInputPorts=2
  Scope2 : Scope  NumInputPorts=2
  Scope3 : Scope  NumInputPorts=2
  cmp_1 : UnitTest_Lib/RoughlyEqual  slope=0.1
  cmp_2 : UnitTest_Lib/RoughlyEqual  slope=0.1
  cmp_3 : UnitTest_Lib/RoughlyEqual  slope=0.1
  result_tws : ToWorkspace  VariableName=spec_result_001
  tws_1 : ToWorkspace  VariableName=spec_req_001_001
  tws_2 : ToWorkspace  VariableName=spec_req_001_002
  tws_3 : ToWorkspace  VariableName=spec_req_001_003
  result : Outport
  wires:
  sig_Req_Bus/1 -> BS_Req/1
  sig_Result_Bus/1 -> BS_Result/1
  AndN/1 -> result/1, result_tws/1
  BS_Req/1 -> cmp_1/1, Scope1/1  "<testSig_PthLead_trqInrCurr>"
  BS_Result/1 -> cmp_1/2, Scope1/2  "<PthLead_trqInrCurr>"
  cmp_1/1 -> Bitwise_And1/1
  Bitwise_And1/1 -> tws_1/1, AndN/1, Scope/1
  BS_Req/2 -> cmp_2/1, Scope2/1  "<testSig_PthLead_trqInrLead>"
  BS_Result/2 -> cmp_2/2, Scope2/2  "<PthLead_trqInrLead>"
  cmp_2/1 -> Bitwise_And2/1
  Bitwise_And2/1 -> tws_2/1, AndN/2, Scope/2
  BS_Req/3 -> cmp_3/1, Scope3/1  "<testSig_PthLead_stActvMonLim>"
  BS_Result/3 -> cmp_3/2, Scope3/2  "<PthLead_stActvMonLim>"
  cmp_3/1 -> Bitwise_And3/1
  Bitwise_And3/1 -> tws_3/1, AndN/3, Scope/3

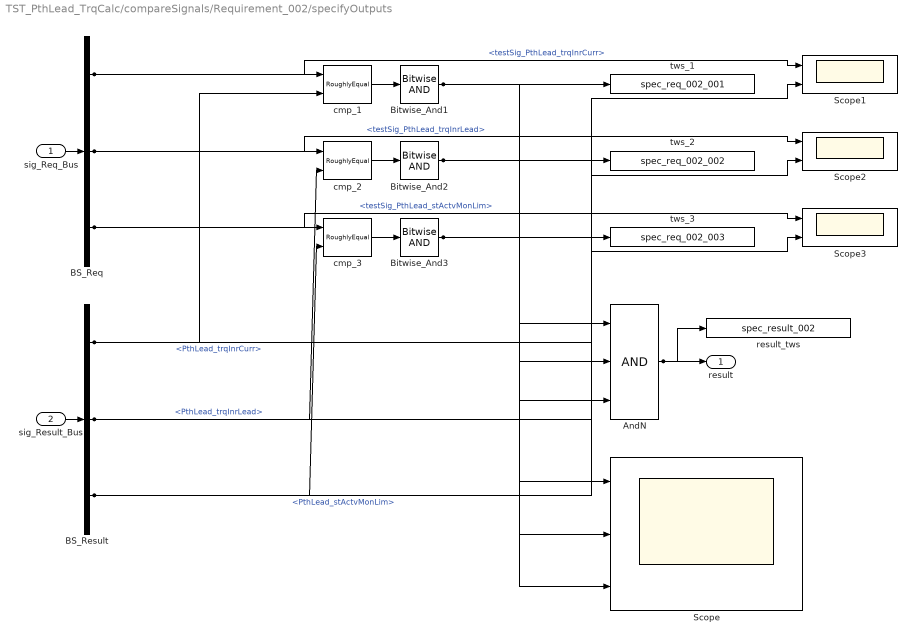
== system TST_PthLead_TrqCalc/compareSignals/Requirement_002/specifyOutputs ==
  sig_Req_Bus : Inport
  sig_Result_Bus : Inport  Port=2
  AndN : Logic  Inputs=3
  BS_Req : BusSelector  OutputSignals=testSig_PthLead_trqInrCurr,testSig_PthLead_trqInrLead,testSig_PthLead_stActvMonLim
  BS_Result : BusSelector  OutputSignals=PthLead_trqInrCurr,PthLead_trqInrLead,PthLead_stActvMonLim
  Bitwise_And1 : simulink/Logic and Bit Operations/Bitwise Operator  logicop=AND  UseBitMask=off  BitMask=bin2dec('11011001')  BitMaskRealWorld=Stored Integer
  Bitwise_And2 : simulink/Logic and Bit Operations/Bitwise Operator  logicop=AND  UseBitMask=off  BitMask=bin2dec('11011001')  BitMaskRealWorld=Stored Integer
  Bitwise_And3 : simulink/Logic and Bit Operations/Bitwise Operator  logicop=AND  UseBitMask=off  BitMask=bin2dec('11011001')  BitMaskRealWorld=Stored Integer
  Scope : Scope  NumInputPorts=3
  Scope1 : Scope  NumInputPorts=2
  Scope2 : Scope  NumInputPorts=2
  Scope3 : Scope  NumInputPorts=2
  cmp_1 : UnitTest_Lib/RoughlyEqual  slope=0.1
  cmp_2 : UnitTest_Lib/RoughlyEqual  slope=0.1
  cmp_3 : UnitTest_Lib/RoughlyEqual  slope=0.1
  result_tws : ToWorkspace  VariableName=spec_result_002
  tws_1 : ToWorkspace  VariableName=spec_req_002_001
  tws_2 : ToWorkspace  VariableName=spec_req_002_002
  tws_3 : ToWorkspace  VariableName=spec_req_002_003
  result : Outport
  wires:
  sig_Req_Bus/1 -> BS_Req/1
  sig_Result_Bus/1 -> BS_Result/1
  AndN/1 -> result/1, result_tws/1
  BS_Req/1 -> cmp_1/1, Scope1/1  "<testSig_PthLead_trqInrCurr>"
  BS_Result/1 -> cmp_1/2, Scope1/2  "<PthLead_trqInrCurr>"
  cmp_1/1 -> Bitwise_And1/1
  Bitwise_And1/1 -> tws_1/1, AndN/1, Scope/1
  BS_Req/2 -> cmp_2/1, Scope2/1  "<testSig_PthLead_trqInrLead>"
  BS_Result/2 -> cmp_2/2, Scope2/2  "<PthLead_trqInrLead>"
  cmp_2/1 -> Bitwise_And2/1
  Bitwise_And2/1 -> tws_2/1, AndN/2, Scope/2
  BS_Req/3 -> cmp_3/1, Scope3/1  "<testSig_PthLead_stActvMonLim>"
  BS_Result/3 -> cmp_3/2, Scope3/2  "<PthLead_stActvMonLim>"
  cmp_3/1 -> Bitwise_And3/1
  Bitwise_And3/1 -> tws_3/1, AndN/3, Scope/3

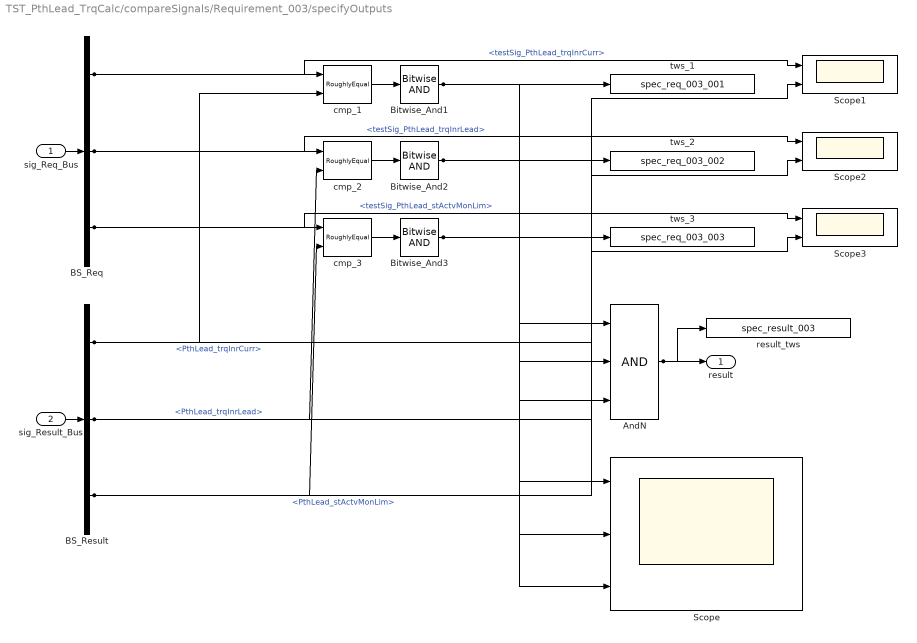
== system TST_PthLead_TrqCalc/compareSignals/Requirement_003/specifyOutputs ==
  sig_Req_Bus : Inport
  sig_Result_Bus : Inport  Port=2
  AndN : Logic  Inputs=3
  BS_Req : BusSelector  OutputSignals=testSig_PthLead_trqInrCurr,testSig_PthLead_trqInrLead,testSig_PthLead_stActvMonLim
  BS_Result : BusSelector  OutputSignals=PthLead_trqInrCurr,PthLead_trqInrLead,PthLead_stActvMonLim
  Bitwise_And1 : simulink/Logic and Bit Operations/Bitwise Operator  logicop=AND  UseBitMask=off  BitMask=bin2dec('11011001')  BitMaskRealWorld=Stored Integer
  Bitwise_And2 : simulink/Logic and Bit Operations/Bitwise Operator  logicop=AND  UseBitMask=off  BitMask=bin2dec('11011001')  BitMaskRealWorld=Stored Integer
  Bitwise_And3 : simulink/Logic and Bit Operations/Bitwise Operator  logicop=AND  UseBitMask=off  BitMask=bin2dec('11011001')  BitMaskRealWorld=Stored Integer
  Scope : Scope  NumInputPorts=3
  Scope1 : Scope  NumInputPorts=2
  Scope2 : Scope  NumInputPorts=2
  Scope3 : Scope  NumInputPorts=2
  cmp_1 : UnitTest_Lib/RoughlyEqual  slope=0.1
  cmp_2 : UnitTest_Lib/RoughlyEqual  slope=0.1
  cmp_3 : UnitTest_Lib/RoughlyEqual  slope=0.1
  result_tws : ToWorkspace  VariableName=spec_result_003
  tws_1 : ToWorkspace  VariableName=spec_req_003_001
  tws_2 : ToWorkspace  VariableName=spec_req_003_002
  tws_3 : ToWorkspace  VariableName=spec_req_003_003
  result : Outport
  wires:
  sig_Req_Bus/1 -> BS_Req/1
  sig_Result_Bus/1 -> BS_Result/1
  AndN/1 -> result/1, result_tws/1
  BS_Req/1 -> cmp_1/1, Scope1/1  "<testSig_PthLead_trqInrCurr>"
  BS_Result/1 -> cmp_1/2, Scope1/2  "<PthLead_trqInrCurr>"
  cmp_1/1 -> Bitwise_And1/1
  Bitwise_And1/1 -> tws_1/1, AndN/1, Scope/1
  BS_Req/2 -> cmp_2/1, Scope2/1  "<testSig_PthLead_trqInrLead>"
  BS_Result/2 -> cmp_2/2, Scope2/2  "<PthLead_trqInrLead>"
  cmp_2/1 -> Bitwise_And2/1
  Bitwise_And2/1 -> tws_2/1, AndN/2, Scope/2
  BS_Req/3 -> cmp_3/1, Scope3/1  "<testSig_PthLead_stActvMonLim>"
  BS_Result/3 -> cmp_3/2, Scope3/2  "<PthLead_stActvMonLim>"
  cmp_3/1 -> Bitwise_And3/1
  Bitwise_And3/1 -> tws_3/1, AndN/3, Scope/3
